simulink model "problem_6"  (R2020b)
settings: Solver=VariableStepAuto  StartTime=0.0  StopTime=10.0  RelTol=1e-3
settings Model: Creator=k.Raviteja  LastModifiedBy=k.Raviteja

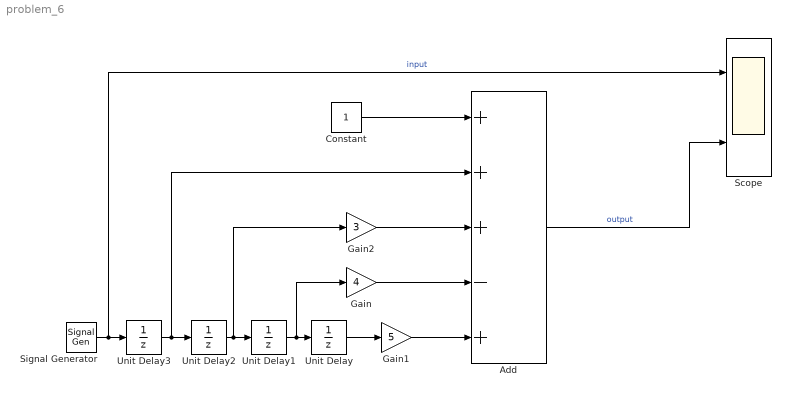
== system problem_6 ==
  Add : Sum  Inputs=+++-+
  Constant : Constant
  Gain : Gain  Gain=4
  Gain1 : Gain  Gain=5
  Gain2 : Gain  Gain=3
  Scope : Scope  NumInputPorts=2
  Signal Generator : SignalGenerator  WaveForm=random  Amplitude=1.5  Units=rad/sec
  Unit Delay{,1..3} (4 alike) : UnitDelay  SampleTime=-1  HasFrameUpgradeWarning=on
  wires:
  Signal Generator/1 -> Scope/1, Unit Delay3/1  "input"
  Unit Delay3/1 -> Add/2, Unit Delay2/1
  Unit Delay2/1 -> Gain2/1, Unit Delay1/1
  Unit Delay1/1 -> Gain/1, Unit Delay/1
  Constant/1 -> Add/1
  Unit Delay/1 -> Gain1/1
  Gain1/1 -> Add/5
  Gain2/1 -> Add/3
  Gain/1 -> Add/4
  Add/1 -> Scope/2  "output"
